simulink model "metareasoning"  (R2020a)
settings: Solver=FixedStepAuto  StartTime=0.0  StopTime=1000  FixedStep=0.5  RelTol=1e-3
PreLoadFcn:
  | Metareasoningpreloadfcn
InitFcn:
  | MetareasoningInitFcn
StopFcn:
  | trajectory_plot
values from neighbouring files (symbols this model uses):
  Clmax = 2.0    (= 2)    [Metareasoningpreloadfcn.m]
  Clmin = -.5    (= -0.5)    [Metareasoningpreloadfcn.m]
  g = 9.81    [Metareasoningpreloadfcn.m]
  goal_pos = [9000, 1E6, 0; -1E6, 23150+9000, 0]    [MetareasoningInitFcn.m]
  LOS_m = 9260    [Metareasoningpreloadfcn.m]
  num_ac = 2    [MetareasoningInitFcn.m]
  omega_chi = .2    (= 0.2)    [Metareasoningpreloadfcn.m]
  omega_gamma = .2    (= 0.2)    [Metareasoningpreloadfcn.m]
  omega_v = .3    (= 0.3)    [Metareasoningpreloadfcn.m]
  rho = 1.225    [Metareasoningpreloadfcn.m]
  S = 37.161    [Metareasoningpreloadfcn.m]
  tau_b = .5    (= 0.5)    [Metareasoningpreloadfcn.m]
  tau_n = .5    (= 0.5)    [Metareasoningpreloadfcn.m]
  tau_t = 1    [Metareasoningpreloadfcn.m]
  thrust_ic = 0.5*rho.*vel_ic.^2*S.*Cd    [MetareasoningInitFcn.m]
  Tmax = 25600*4.44822    (= 113874.432)    [Metareasoningpreloadfcn.m]
  W = 14515    [Metareasoningpreloadfcn.m]
undefined symbols (not defined in the file or in its folder): turnangles
libraries: asbswarm_lib x2, aerolibptmass x2, simulink x1
(part 1 of 3)
settings Model: Creator=Aidan  LastModifiedBy=Aidan

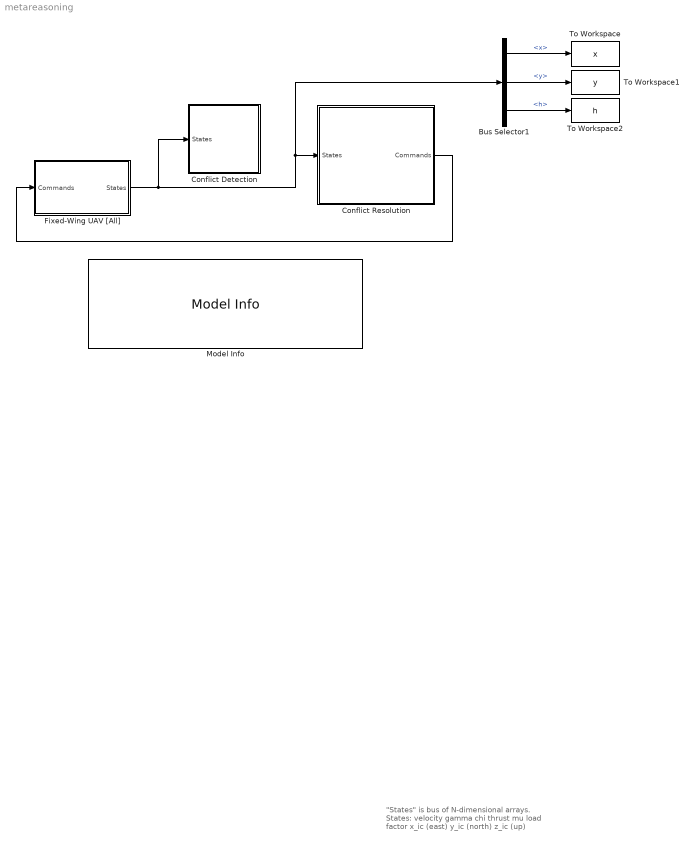
== system metareasoning ==
  note: "States" is bus of N-dimensional arrays.
      |
      | States:
      | velocity
      | gamma
      | chi
      | thrust
      | mu
      | load factor
      | x_ic (east)
      | y_ic (north)
      | z_ic (up)
  Bus Selector1 : BusSelector  OutputSignals=x,y,h
  Conflict Detection : Subsystem
      mask Display: image('C:\Users\Aidan\Downloads\exclamation_mark.png'); % Use "Edit Image" on toolstrip to change.
  Conflict Resolution : Subsystem
  Fixed-Wing UAV [All] : Subsystem
  Model Info : simulink/Model-Wide Utilities/Model Info  Frame=on  DisplayStringWithTags=|  HorizontalTextAlignment=Center  LeftAlignmentValue=0.5
      | Aidan Wallace
      | University of Maryland, College Park
      | 
      | This multiple-aircraft model is used to demonstrate the performance 
      | of various conflict detection and resolution methods for winged aircraft.
      | 
      | Fixed-Wing UAV and DynInversionControl blocks modified from Simulink
      | example model 'asbswarm'
      | 
      | %<LastModificationDate>
  To Workspace : ToWorkspace  VariableName=x  SaveFormat=Timeseries  SampleTime=-1
  To Workspace1 : ToWorkspace  VariableName=y  SaveFormat=Timeseries  SampleTime=-1
  To Workspace2 : ToWorkspace  VariableName=h  SaveFormat=Timeseries  SampleTime=-1
  wires:
  Bus Selector1/2 -> To Workspace1/1  "<y>"
  Bus Selector1/1 -> To Workspace/1  "<x>"
  Bus Selector1/3 -> To Workspace2/1  "<h>"
  Fixed-Wing UAV [All]/1(States) -> Bus Selector1/1, Conflict Resolution/1(States), Conflict Detection/1(States)
  Conflict Resolution/1(Commands) -> Fixed-Wing UAV [All]/1(Commands)

== system metareasoning/Conflict Detection ==
  States : Inport
  Bus Selector : BusSelector  OutputSignals=Velocity,chi,x,y
  State-Based Conflict Detection (Single Agent) : Subsystem  TreatAsAtomicUnit=on
  To Workspace : ToWorkspace  VariableName=tlos  SaveFormat=Timeseries  SampleTime=-1
  To Workspace1 : ToWorkspace  VariableName=tcpa  SaveFormat=Timeseries  SampleTime=-1
  wires:
  Bus Selector/2 -> State-Based Conflict Detection (Single Agent)/6(chi [all]), State-Based Conflict Detection (Single Agent)/2(chi (own))  "<chi>"
  Bus Selector/1 -> State-Based Conflict Detection (Single Agent)/1(Velocity (own)), State-Based Conflict Detection (Single Agent)/5(velocity [all])  "<Velocity>"
  Bus Selector/4 -> State-Based Conflict Detection (Single Agent)/8(y [all]), State-Based Conflict Detection (Single Agent)/4(y (own))  "<y>"
  State-Based Conflict Detection (Single Agent)/1(tlos) -> To Workspace/1  "tlos"
  Bus Selector/3 -> State-Based Conflict Detection (Single Agent)/7(x [all]), State-Based Conflict Detection (Single Agent)/3(x (own))  "<x>"
  States/1 -> Bus Selector/1
  State-Based Conflict Detection (Single Agent)/2(tcpa) -> To Workspace1/1

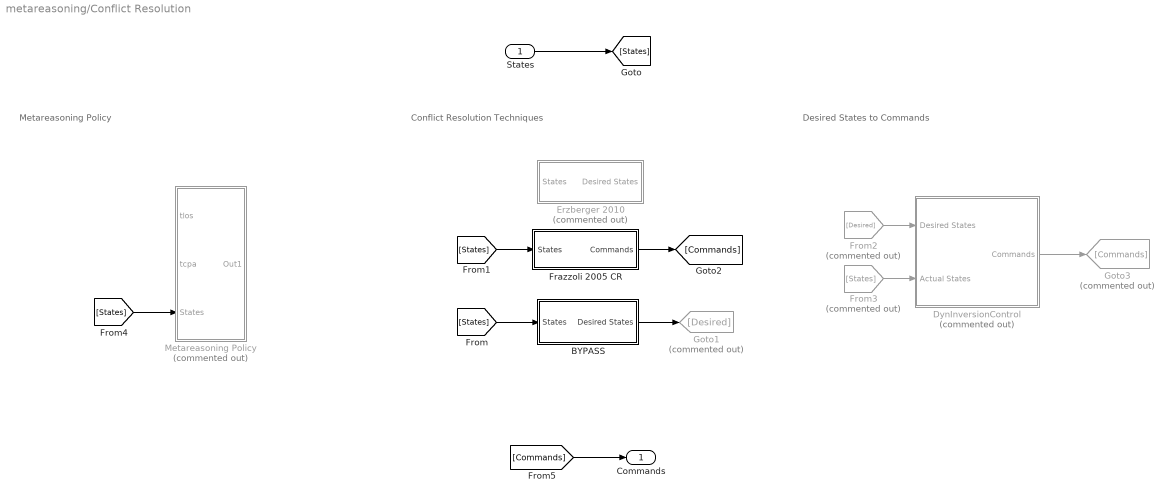
== system metareasoning/Conflict Resolution ==
  note: Desired States to Commands
  note: Conflict Resolution Techniques
  note: Metareasoning Policy
  States : Inport
  BYPASS : Subsystem
  DynInversionControl : Subsystem  Commented=on
  Erzberger 2010 : Subsystem  Commented=on
  Frazzoli 2005 CR : Subsystem
  From2 : From  Commented=on  GotoTag=Desired
  From3 : From  Commented=on  GotoTag=States
  Goto1 : Goto  Commented=on  GotoTag=Desired
  Goto3 : Goto  Commented=on  GotoTag=Commands
  Metareasoning Policy : Subsystem  Commented=on
  Commands : Outport
  wires:
  DynInversionControl/1(Commands) -> Goto3/1
  BYPASS/1(Desired States) -> Goto1/1
  States/1 -> [States]
  [States] -> BYPASS/1(States)
  [States] -> Frazzoli 2005 CR/1(States)
  From2/1 -> DynInversionControl/1(Desired States)
  From3/1 -> DynInversionControl/2(Actual States)
  [States] -> Metareasoning Policy/3(States)
  Frazzoli 2005 CR/1(Commands) -> [Commands]
  [Commands] -> Commands/1

== system metareasoning/Fixed-Wing UAV [All] ==
  Commands : Inport
  6DOF Point Mass (Coordinated Flight) : aerolibptmass/6th Order Point Mass (Coordinated Flight)  units=Metric (MKS)  gamma0=gamma_ic  chi0=chi_ic  V0=vel_ic  x0=x0  y0=y0  h0=h0  mass0=W/g
      settings: SourceProductBaseCode=AE
  6DOF Point Mass Forces (Coordinated Flight) : aerolibptmass/6th Order Point Mass Forces (Coordinated Flight)
      settings: SourceProductBaseCode=AE
  "Commands " : InportShadow
  EOM : Subsystem
  Integrator : Integrator  InitialCondition=[thrust_ic; zeros(1,num_ac); ones(1,num_ac)]
  Subsystem1 : Subsystem
  "V, gamma, chi2" : BusSelector  OutputSignals=gamma
  "V, gamma, chi4" : BusSelector  OutputSignals=mu
  alpha : Constant  Value=0
  makebus1 : Subsystem
  States : Outport  VectorParamsAs1DForOutWhenUnconnected=off
  wires:
  EOM/1(State Rates) -> Integrator/1
  Integrator/1 -> makebus1/1(In1)
  6DOF Point Mass Forces (Coordinated Flight)/2 -> 6DOF Point Mass (Coordinated Flight)/2
  6DOF Point Mass (Coordinated Flight)/3 -> makebus1/4(Velocity)
  6DOF Point Mass (Coordinated Flight)/1 -> makebus1/2(gamma)
  6DOF Point Mass Forces (Coordinated Flight)/1 -> 6DOF Point Mass (Coordinated Flight)/1
  6DOF Point Mass (Coordinated Flight)/2 -> makebus1/3(chi)
  6DOF Point Mass (Coordinated Flight)/6 -> makebus1/7(h)
  makebus1/1(Out2) -> States/1, "V, gamma, chi4"/1, "V, gamma, chi2"/1, Subsystem1/2(States), EOM/1(States)
  6DOF Point Mass Forces (Coordinated Flight)/3 -> 6DOF Point Mass (Coordinated Flight)/3
  Subsystem1/4(Thrust) -> 6DOF Point Mass Forces (Coordinated Flight)/4
  Subsystem1/2(Drag) -> 6DOF Point Mass Forces (Coordinated Flight)/2
  Subsystem1/1(Lift) -> 6DOF Point Mass Forces (Coordinated Flight)/1
  Subsystem1/3(Weight) -> 6DOF Point Mass Forces (Coordinated Flight)/3
  alpha/1 -> 6DOF Point Mass Forces (Coordinated Flight)/7
  "V, gamma, chi4"/1 -> 6DOF Point Mass Forces (Coordinated Flight)/6  "<mu>"
  6DOF Point Mass (Coordinated Flight)/4 -> makebus1/5(x)
  6DOF Point Mass (Coordinated Flight)/5 -> makebus1/6(y)
  "Commands "/1 -> Subsystem1/1(Cmd)
  Commands/1 -> EOM/2(Commands)
  "V, gamma, chi2"/1 -> 6DOF Point Mass Forces (Coordinated Flight)/5  "<gamma>"

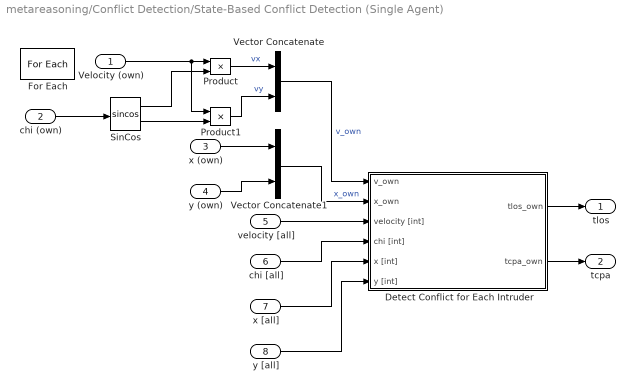
== system metareasoning/Conflict Detection/State-Based Conflict Detection (Single Agent) ==
  Velocity (own) : Inport  Partition=on  PartitionDimension=1  PartitionWidth=1  PartitionOffset=0
  chi (own) : Inport  Port=2  Partition=on  PartitionDimension=1  PartitionWidth=1  PartitionOffset=0
  x (own) : Inport  Port=3  Partition=on  PartitionDimension=1  PartitionWidth=1  PartitionOffset=0
  y (own) : Inport  Port=4  Partition=on  PartitionDimension=1  PartitionWidth=1  PartitionOffset=0
  velocity [all] : Inport  Port=5
  chi [all] : Inport  Port=6
  x [all] : Inport  Port=7
  y [all] : Inport  Port=8
  Detect Conflict for Each Intruder : Subsystem  TreatAsAtomicUnit=on
  For Each : ForEach  DisableCoverage=on
  Product : Product
  Product1 : Product
  SinCos : Trigonometry  Operator=sincos
  Vector Concatenate : Concatenate
  Vector Concatenate1 : Concatenate
  tlos : Outport  ConcatenationDimension=1
  tcpa : Outport  Port=2  ConcatenationDimension=1
  wires:
  Product1/1 -> Vector Concatenate/2  "vy"
  SinCos/1 -> Product/2
  Detect Conflict for Each Intruder/2(tcpa_own) -> tcpa/1
  Vector Concatenate/1 -> Detect Conflict for Each Intruder/1(v_own)  "v_own"
  Vector Concatenate1/1 -> Detect Conflict for Each Intruder/2(x_own)  "x_own"
  Detect Conflict for Each Intruder/1(tlos_own) -> tlos/1
  chi (own)/1 -> SinCos/1
  chi [all]/1 -> Detect Conflict for Each Intruder/4(chi [int])
  y [all]/1 -> Detect Conflict for Each Intruder/6(y [int])
  x [all]/1 -> Detect Conflict for Each Intruder/5(x [int])
  velocity [all]/1 -> Detect Conflict for Each Intruder/3(velocity [int])
  Product/1 -> Vector Concatenate/1  "vx"
  SinCos/2 -> Product1/2
  y (own)/1 -> Vector Concatenate1/2
  x (own)/1 -> Vector Concatenate1/1
  Velocity (own)/1 -> Product/1, Product1/1

== system metareasoning/Conflict Resolution/BYPASS ==
  States : Inport
  Bus Creator : BusCreator  Inputs=3
  Bus Selector : BusSelector  OutputSignals=Velocity,gamma,chi
  Sum : Sum  Inputs=|++
  Sum1 : Sum  Inputs=|++
  Sum2 : Sum  Inputs=|++
  Zero : Constant  Value=0  OutDataTypeStr=Inherit: Inherit via back propagation
  Desired States : Outport
  wires:
  States/1 -> Bus Selector/1
  Bus Creator/1 -> Desired States/1
  Bus Selector/1 -> Sum/1  "<Velocity>"
  Bus Selector/2 -> Sum1/1  "<gamma>"
  Zero/1 -> Sum2/2, Sum1/2, Sum/2
  Bus Selector/3 -> Sum2/1  "<chi>"
  Sum2/1 -> Bus Creator/3  "chi_desired"
  Sum1/1 -> Bus Creator/2  "gamma_desired"
  Sum/1 -> Bus Creator/1  "Velocity_desired"

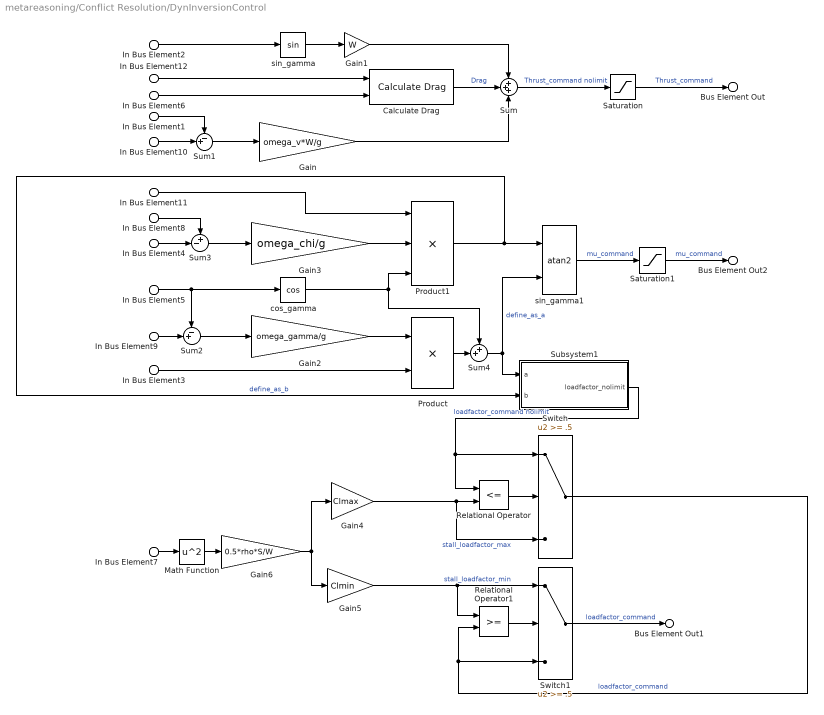
== system metareasoning/Conflict Resolution/DynInversionControl ==
  In Bus Element8 : Inport  PortName=Desired States  Element=chi_desired
  In Bus Element9 : Inport  PortName=Desired States  Element=gamma_desired
  In Bus Element10 : Inport  PortName=Desired States  Element=Velocity_desired
  In Bus Element{1,3,7,11..12} (5 alike) : Inport  Port=2  PortName=Actual States  Element=Velocity
  In Bus Element5 : Inport  Port=2  PortName=Actual States  Element=gamma
  In Bus Element2 : Inport  Port=2  PortName=Actual States  Element=gamma
  In Bus Element4 : Inport  Port=2  PortName=Actual States  Element=chi
  In Bus Element6 : Inport  Port=2  PortName=Actual States  Element=loadfactor
  Calculate Drag : asbswarm_lib/Calculate Drag  SystemSampleTime=-1  Latency=0  AutoFrameSizeCalculation=off
      settings: SourceProductBaseCode=AE
  Gain : Gain  Gain=omega_v*W/g  SaturateOnIntegerOverflow=on  OutDataTypeStr=Inherit: Same as input  ParamDataTypeStr=Inherit: Same as input
  Gain1 : Gain  Gain=W  SaturateOnIntegerOverflow=on  OutDataTypeStr=Inherit: Same as input  ParamDataTypeStr=Inherit: Same as input
  Gain2 : Gain  Gain=omega_gamma/g  SaturateOnIntegerOverflow=on  OutDataTypeStr=Inherit: Same as input  ParamDataTypeStr=Inherit: Same as input
  Gain3 : Gain  Gain=omega_chi/g  SaturateOnIntegerOverflow=on  OutDataTypeStr=Inherit: Same as input  ParamDataTypeStr=Inherit: Same as input
  Gain4 : Gain  Gain=Clmax  SaturateOnIntegerOverflow=on  OutDataTypeStr=Inherit: Same as input  ParamDataTypeStr=Inherit: Same as input
  Gain5 : Gain  Gain=Clmin  SaturateOnIntegerOverflow=on  OutDataTypeStr=Inherit: Same as input  ParamDataTypeStr=Inherit: Same as input
  Gain6 : Gain  Gain=0.5*rho*S/W  SaturateOnIntegerOverflow=on  OutDataTypeStr=Inherit: Same as input  ParamDataTypeStr=Inherit: Same as input
  Math Function : Math  Operator=square  SignedPower=on  SaturateOnIntegerOverflow=on
  Product : Product  InputSameDT=on  SaturateOnIntegerOverflow=on  OutDataTypeStr=Inherit: Same as first input
  Product1 : Product  Inputs=3  InputSameDT=on  SaturateOnIntegerOverflow=on  OutDataTypeStr=Inherit: Same as first input
  Relational Operator : RelationalOperator  Operator=<=  RndMeth=Nearest  InputSameDT=on
  Relational Operator1 : RelationalOperator  RndMeth=Nearest  InputSameDT=on
  Saturation : Saturate  UpperLimit=Tmax  LowerLimit=0
  Saturation1 : Saturate  UpperLimit=pi/2  LowerLimit=-pi/2
  Subsystem1 : Subsystem
  Sum : Sum  Inputs=+++  InputSameDT=on  SaturateOnIntegerOverflow=on  OutDataTypeStr=Inherit: Same as first input
  Sum1 : Sum  Inputs=-+|  InputSameDT=on  SaturateOnIntegerOverflow=on  OutDataTypeStr=Inherit: Same as first input
  Sum2 : Sum  Inputs=-+|  InputSameDT=on  SaturateOnIntegerOverflow=on  OutDataTypeStr=Inherit: Same as first input
  Sum3 : Sum  Inputs=+-|  InputSameDT=on  SaturateOnIntegerOverflow=on  OutDataTypeStr=Inherit: Same as first input
  Sum4 : Sum  Inputs=++|  InputSameDT=on  SaturateOnIntegerOverflow=on  OutDataTypeStr=Inherit: Same as first input
  Switch : Switch  Threshold=.5  SaturateOnIntegerOverflow=on  InputSameDT=on
  Switch1 : Switch  Threshold=.5  SaturateOnIntegerOverflow=on  InputSameDT=on
  cos_gamma : Trigonometry  Operator=cos
  sin_gamma : Trigonometry
  sin_gamma1 : Trigonometry  Operator=atan2
  Bus Element Out : Outport  VectorParamsAs1DForOutWhenUnconnected=off  PortName=Commands  Element=Thrust_command
  Bus Element Out1 : Outport  VectorParamsAs1DForOutWhenUnconnected=off  PortName=Commands  Element=loadfactor_command
  Bus Element Out2 : Outport  VectorParamsAs1DForOutWhenUnconnected=off  PortName=Commands  Element=mu_command
  wires:
  In Bus Element9/1 -> Sum2/2
  In Bus Element6/1 -> Calculate Drag/2
  In Bus Element1/1 -> Sum1/1
  In Bus Element10/1 -> Sum1/2
  Sum1/1 -> Gain/1
  Calculate Drag/1 -> Sum/2  "Drag"
  Gain/1 -> Sum/3
  In Bus Element2/1 -> sin_gamma/1
  sin_gamma/1 -> Gain1/1
  Gain1/1 -> Sum/1
  Sum/1 -> Saturation/1  "Thrust_command nolimit"
  In Bus Element5/1 -> Sum2/1, cos_gamma/1
  In Bus Element8/1 -> Sum3/1
  In Bus Element4/1 -> Sum3/2
  Sum2/1 -> Gain2/1
  Gain2/1 -> Product/1
  In Bus Element3/1 -> Product/2
  Product/1 -> Sum4/2
  cos_gamma/1 -> Product1/3, Sum4/1
  Sum4/1 -> Subsystem1/1(a), sin_gamma1/2  "define_as_a"
  Sum3/1 -> Gain3/1
  Product1/1 -> Subsystem1/2(b), sin_gamma1/1  "define_as_b"
  sin_gamma1/1 -> Saturation1/1  "mu_command"
  Subsystem1/1(loadfactor_nolimit) -> Switch/1, Relational Operator/1  "loadfactor_command nolimit"
  Saturation/1 -> Bus Element Out/1  "Thrust_command"
  In Bus Element7/1 -> Math Function/1
  Gain3/1 -> Product1/2
  Gain4/1 -> Switch/3, Relational Operator/2  "stall_loadfactor_max"
  Relational Operator/1 -> Switch/2
  Math Function/1 -> Gain6/1
  Saturation1/1 -> Bus Element Out2/1  "mu_command"
  Gain5/1 -> Switch1/1, Relational Operator1/1  "stall_loadfactor_min"
  Switch/1 -> Switch1/3, Relational Operator1/2  "loadfactor_command"
  Relational Operator1/1 -> Switch1/2
  Switch1/1 -> Bus Element Out1/1  "loadfactor_command"
  In Bus Element11/1 -> Product1/1
  In Bus Element12/1 -> Calculate Drag/1
  Gain6/1 -> Gain4/1, Gain5/1

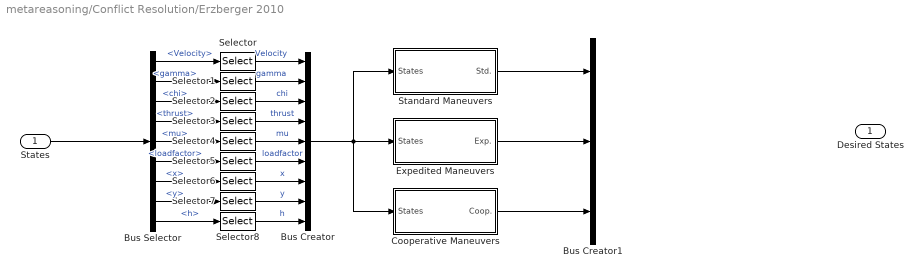
== system metareasoning/Conflict Resolution/Erzberger 2010 ==
  States : Inport
  Bus Creator : BusCreator  Inputs=9
  Bus Creator1 : BusCreator  Inputs=3
  Bus Selector : BusSelector  OutputSignals=Velocity,gamma,chi,thrust,mu,loadfactor,x,y,h
  Cooperative Maneuvers : Subsystem
  Expedited Maneuvers : Subsystem
  Selector{,1..8} (9 alike) : Selector  InputPortWidth=num_ac  IndexOptions=Index vector (dialog)  Indices=[1 2]  OutputSizes=1
  Standard Maneuvers : Subsystem
  Desired States : Outport
  wires:
  States/1 -> Bus Selector/1
  Bus Selector/1 -> Selector/1  "<Velocity>"
  Bus Selector/2 -> Selector1/1  "<gamma>"
  Bus Selector/3 -> Selector2/1  "<chi>"
  Bus Selector/4 -> Selector3/1  "<thrust>"
  Bus Selector/5 -> Selector4/1  "<mu>"
  Bus Selector/6 -> Selector5/1  "<loadfactor>"
  Bus Selector/7 -> Selector6/1  "<x>"
  Bus Selector/8 -> Selector7/1  "<y>"
  Bus Selector/9 -> Selector8/1  "<h>"
  Selector/1 -> Bus Creator/1  "Velocity"
  Selector1/1 -> Bus Creator/2  "gamma"
  Selector2/1 -> Bus Creator/3  "chi"
  Selector3/1 -> Bus Creator/4  "thrust"
  Selector4/1 -> Bus Creator/5  "mu"
  Selector5/1 -> Bus Creator/6  "loadfactor"
  Selector6/1 -> Bus Creator/7  "x"
  Selector7/1 -> Bus Creator/8  "y"
  Selector8/1 -> Bus Creator/9  "h"
  Bus Creator/1 -> Standard Maneuvers/1(States), Cooperative Maneuvers/1(States), Expedited Maneuvers/1(States)
  Standard Maneuvers/1(Std.) -> Bus Creator1/1
  Cooperative Maneuvers/1(Coop.) -> Bus Creator1/3
  Expedited Maneuvers/1(Exp.) -> Bus Creator1/2

== system metareasoning/Conflict Resolution/Frazzoli 2005 CR ==
  States : Inport
  Bus Selector : BusSelector  OutputSignals=x,y,chi,Velocity,thrust
  Constant : Constant  Value=goal_pos
  Single-Agent Planning : Subsystem  TreatAsAtomicUnit=on
  Bus Element Out : Outport  PortName=Commands  Element=Thrust_command
  Bus Element Out1 : Outport  PortName=Commands  Element=mu_command
  Bus Element Out2 : Outport  PortName=Commands  Element=loadfactor_command
  wires:
  States/1 -> Bus Selector/1
  Bus Selector/1 -> Single-Agent Planning/5(x [all]), Single-Agent Planning/1(<x>)  "<x>"
  Bus Selector/2 -> Single-Agent Planning/6(y [all]), Single-Agent Planning/2(<y>)  "<y>"
  Bus Selector/3 -> Single-Agent Planning/7(chi [all]), Single-Agent Planning/3(<chi>)  "<chi>"
  Single-Agent Planning/1(Thrust_command) -> Bus Element Out/1
  Constant/1 -> Single-Agent Planning/8(goal_pos)
  Bus Selector/4 -> Single-Agent Planning/4(Velocity)  "<Velocity>"
  Bus Selector/5 -> Single-Agent Planning/9(Thrust)  "<thrust>"
  Single-Agent Planning/2(mu_command) -> Bus Element Out1/1
  Single-Agent Planning/3(loadfactor_command) -> Bus Element Out2/1

== system metareasoning/Conflict Resolution/Metareasoning Policy ==
  tlos : Inport
  tcpa : Inport  Port=2
  States : Inport  Port=3
  Out1 : Outport
  wires:
  tlos/1 -> Out1/1

== system metareasoning/Fixed-Wing UAV [All]/EOM ==
  States : Inport
  Commands : Inport  Port=2
  Math Function : Math  Operator=transpose  SignedPower=on  SaturateOnIntegerOverflow=on
  Matrix Concatenation : Concatenate  NumInputs=3  Mode=Multidimensional array  ConcatenateDimension=2
  "[thrust_dot mu_dot loadfactor_dot]" : Subsystem
  State Rates : Outport  VectorParamsAs1DForOutWhenUnconnected=off
  wires:
  Commands/1 -> "[thrust_dot mu_dot loadfactor_dot]"/1(Commands)
  States/1 -> "[thrust_dot mu_dot loadfactor_dot]"/2(States)
  "[thrust_dot mu_dot loadfactor_dot]"/2(mu_dot) -> Matrix Concatenation/2
  "[thrust_dot mu_dot loadfactor_dot]"/1(thrust_dot) -> Matrix Concatenation/1
  "[thrust_dot mu_dot loadfactor_dot]"/3(loadfactor_dot) -> Matrix Concatenation/3
  Math Function/1 -> State Rates/1
  Matrix Concatenation/1 -> Math Function/1

== system metareasoning/Fixed-Wing UAV [All]/Subsystem1 ==
  Bus Element In2 : Inport  PortName=Cmd  Element=Thrust_command
  Bus Element In : Inport  Port=2  PortName=States  Element=loadfactor
  Bus Element In1 : Inport  Port=2  PortName=States  Element=loadfactor
  Bus Element In3 : Inport  Port=2  PortName=States  Element=Velocity
  Calculate Drag : asbswarm_lib/Calculate Drag  SystemSampleTime=-1  Latency=0  AutoFrameSizeCalculation=off
      settings: SourceProductBaseCode=AE
  Constant : Constant  Value=W
  Product1 : Product  RndMeth=Zero
  Lift : Outport  VectorParamsAs1DForOutWhenUnconnected=off
  Drag : Outport  Port=2  VectorParamsAs1DForOutWhenUnconnected=off
  Weight : Outport  Port=3  VectorParamsAs1DForOutWhenUnconnected=off
  Thrust : Outport  Port=4  VectorParamsAs1DForOutWhenUnconnected=off
  wires:
  Constant/1 -> Product1/2, Weight/1
  Calculate Drag/1 -> Drag/1
  Bus Element In2/1 -> Thrust/1
  Product1/1 -> Lift/1
  Bus Element In3/1 -> Calculate Drag/1
  Bus Element In/1 -> Calculate Drag/2
  Bus Element In1/1 -> Product1/1

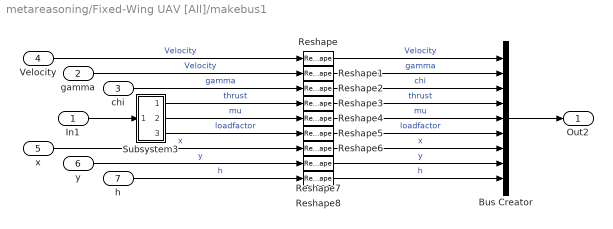
== system metareasoning/Fixed-Wing UAV [All]/makebus1 ==
  In1 : Inport  PortDimensions=[3,num_ac]
  gamma : Inport  Port=2  PortDimensions=[1,num_ac]
  chi : Inport  Port=3  PortDimensions=[1,num_ac]
  Velocity : Inport  Port=4  PortDimensions=[1,num_ac]
  x : Inport  Port=5  PortDimensions=[1,num_ac]
  y : Inport  Port=6  PortDimensions=[1,num_ac]
  h : Inport  Port=7  PortDimensions=[1,num_ac]
  Bus Creator : BusCreator  Inputs=9
  Reshape{,1..8} (9 alike) : Reshape
  Subsystem3 : Subsystem
      mask Display: disp('Select\nRows');
  Out2 : Outport  VectorParamsAs1DForOutWhenUnconnected=off
  wires:
  In1/1 -> Subsystem3/1(In1)
  Reshape8/1 -> Bus Creator/9  "h"
  Reshape7/1 -> Bus Creator/8  "y"
  Reshape6/1 -> Bus Creator/7  "x"
  Reshape5/1 -> Bus Creator/6  "loadfactor"
  Reshape4/1 -> Bus Creator/5  "mu"
  Reshape3/1 -> Bus Creator/4  "thrust"
  Reshape2/1 -> Bus Creator/3  "chi"
  Reshape1/1 -> Bus Creator/2  "gamma"
  Reshape/1 -> Bus Creator/1  "Velocity"
  Bus Creator/1 -> Out2/1
  h/1 -> Reshape8/1  "h"
  y/1 -> Reshape7/1  "y"
  x/1 -> Reshape6/1  "x"
  Subsystem3/3(Out3) -> Reshape5/1  "loadfactor"
  Subsystem3/2(Out2) -> Reshape4/1  "mu"
  Subsystem3/1(Out1) -> Reshape3/1  "thrust"
  chi/1 -> Reshape2/1  "gamma"
  gamma/1 -> Reshape1/1  "Velocity"
  Velocity/1 -> Reshape/1  "Velocity"

== system metareasoning/Conflict Detection/State-Based Conflict Detection (Single Agent)/Detect Conflict for Each Intruder ==
  v_own : Inport
  x_own : Inport  Port=2
  velocity [int] : Inport  Port=3  Partition=on  PartitionDimension=1  PartitionWidth=1  PartitionOffset=0
  chi [int] : Inport  Port=4  Partition=on  PartitionDimension=1  PartitionWidth=1  PartitionOffset=0
  x [int] : Inport  Port=5  Partition=on  PartitionDimension=1  PartitionWidth=1  PartitionOffset=0
  y [int] : Inport  Port=6  Partition=on  PartitionDimension=1  PartitionWidth=1  PartitionOffset=0
  Conflict Detection : MATLAB Function  TreatAsAtomicUnit=on
  Constant : Constant  Value=LOS_m
  For Each : ForEach  DisableCoverage=on
  Product : Product
  Product1 : Product
  SinCos : Trigonometry  Operator=sincos
  Vector Concatenate : Concatenate
  Vector Concatenate1 : Concatenate
  tlos_own : Outport  ConcatenationDimension=2
  tcpa_own : Outport  Port=2  ConcatenationDimension=2
  wires:
  velocity [int]/1 -> Product/1, Product1/1
  Product/1 -> Vector Concatenate/1  "vx"
  x_own/1 -> Conflict Detection/2(x_own)
  Constant/1 -> Conflict Detection/5(LOS_m)
  Conflict Detection/1(tlos) -> tlos_own/1
  chi [int]/1 -> SinCos/1
  y [int]/1 -> Vector Concatenate1/2
  v_own/1 -> Conflict Detection/1(v_own)
  SinCos/1 -> Product/2
  Vector Concatenate/1 -> Conflict Detection/3(v_int)  "v_int"
  SinCos/2 -> Product1/2
  Vector Concatenate1/1 -> Conflict Detection/4(x_int)  "x_int"
  Conflict Detection/2(tcpa) -> tcpa_own/1
  Product1/1 -> Vector Concatenate/2  "vy"
  x [int]/1 -> Vector Concatenate1/1

== system metareasoning/Conflict Resolution/DynInversionControl/Subsystem1 ==
  a : Inport
  b : Inport  Port=2
  Math Function : Math  Operator=square  SignedPower=on  SaturateOnIntegerOverflow=on
  Math Function1 : Math  Operator=square  SignedPower=on  SaturateOnIntegerOverflow=on
  Sqrt : Sqrt  SaturateOnIntegerOverflow=on
  Sum : Sum  Inputs=|++  InputSameDT=on  SaturateOnIntegerOverflow=on  OutDataTypeStr=Inherit: Same as first input
  loadfactor_nolimit : Outport  VectorParamsAs1DForOutWhenUnconnected=off
  wires:
  Sqrt/1 -> loadfactor_nolimit/1
  Math Function1/1 -> Sum/2
  Math Function/1 -> Sum/1
  b/1 -> Math Function1/1
  a/1 -> Math Function/1
  Sum/1 -> Sqrt/1

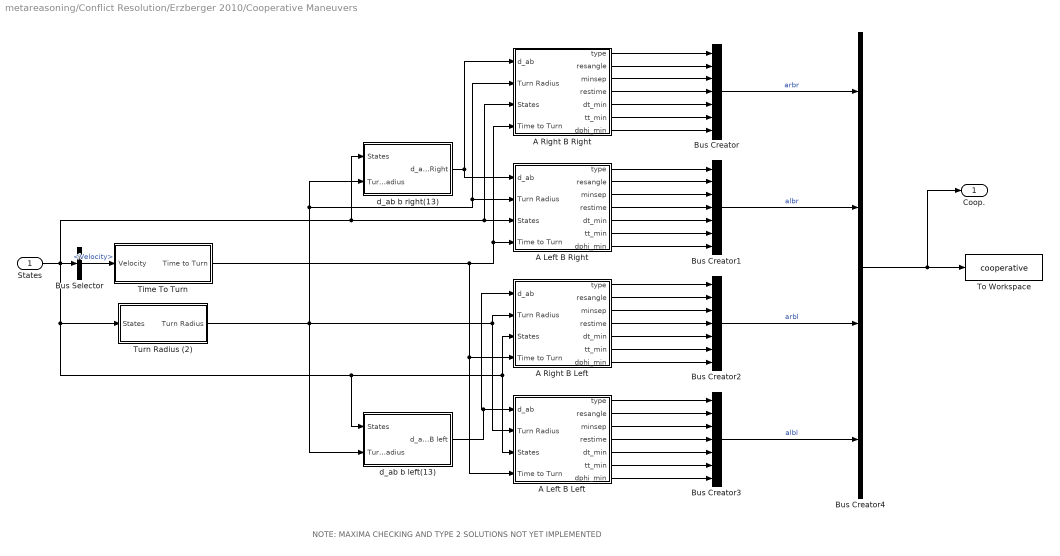
== system metareasoning/Conflict Resolution/Erzberger 2010/Cooperative Maneuvers ==
  note: NOTE: MAXIMA CHECKING AND TYPE 2 SOLUTIONS NOT YET IMPLEMENTED
  States : Inport
  A Left B Left : Subsystem
  A Left B Right : Subsystem
  A Right B Left : Subsystem
  A Right B Right : Subsystem
  Bus Creator{,1..3} (4 alike) : BusCreator  Inputs=7
  Bus Creator4 : BusCreator  Inputs=4
  Bus Selector : BusSelector  OutputSignals=Velocity
  Time To Turn : Subsystem
  To Workspace : ToWorkspace  VariableName=cooperative  SaveFormat=Timeseries  SampleTime=-1
  Turn Radius (2) : Subsystem
  d_ab b left(13) : Subsystem
  d_ab b right(13) : Subsystem
  Coop. : Outport
  wires:
  Bus Selector/1 -> Time To Turn/1(Velocity)  "<Velocity>"
  States/1 -> A Right B Left/3(States), A Left B Left/3(States), d_ab b left(13)/1(States), Turn Radius (2)/1(States), d_ab b right(13)/1(States), A Right B Right/3(States), A Left B Right/3(States), Bus Selector/1
  Time To Turn/1(Time to Turn) -> A Right B Left/4(Time to Turn), A Left B Left/4(Time to Turn), A Left B Right/4(Time to Turn), A Right B Right/4(Time to Turn)
  Turn Radius (2)/1(Turn Radius) -> d_ab b left(13)/2(Turn Radius), A Right B Left/2(Turn Radius), A Left B Left/2(Turn Radius), d_ab b right(13)/2(Turn Radius), A Left B Right/2(Turn Radius), A Right B Right/2(Turn Radius)
  d_ab b right(13)/1(d_ab B Right) -> A Left B Right/1(d_ab), A Right B Right/1(d_ab)
  A Right B Right/2(resangle) -> Bus Creator/2
  A Right B Right/3(minsep) -> Bus Creator/3
  A Right B Right/4(restime) -> Bus Creator/4
  A Right B Right/5(dt_min) -> Bus Creator/5
  A Right B Right/6(tt_min) -> Bus Creator/6
  A Right B Right/7(dphi_min) -> Bus Creator/7
  A Right B Right/1(type) -> Bus Creator/1
  Bus Creator/1 -> Bus Creator4/1  "arbr"
  Bus Creator1/1 -> Bus Creator4/2  "albr"
  Bus Creator2/1 -> Bus Creator4/3  "arbl"
  Bus Creator3/1 -> Bus Creator4/4  "albl"
  Bus Creator4/1 -> Coop./1, To Workspace/1
  A Left B Right/2(resangle) -> Bus Creator1/2
  A Left B Right/1(type) -> Bus Creator1/1
  A Left B Right/3(minsep) -> Bus Creator1/3
  A Left B Right/4(restime) -> Bus Creator1/4
  A Left B Right/5(dt_min) -> Bus Creator1/5
  A Left B Right/6(tt_min) -> Bus Creator1/6
  A Left B Right/7(dphi_min) -> Bus Creator1/7
  A Left B Left/1(type) -> Bus Creator3/1
  A Left B Left/2(resangle) -> Bus Creator3/2
  A Left B Left/3(minsep) -> Bus Creator3/3
  A Left B Left/4(restime) -> Bus Creator3/4
  A Left B Left/5(dt_min) -> Bus Creator3/5
  A Left B Left/6(tt_min) -> Bus Creator3/6
  A Left B Left/7(dphi_min) -> Bus Creator3/7
  d_ab b left(13)/1(d_ab B left) -> A Right B Left/1(d_ab), A Left B Left/1(d_ab)
  A Right B Left/1(type) -> Bus Creator2/1
  A Right B Left/2(resangle) -> Bus Creator2/2
  A Right B Left/3(minsep) -> Bus Creator2/3
  A Right B Left/4(restime) -> Bus Creator2/4
  A Right B Left/5(dt_min) -> Bus Creator2/5
  A Right B Left/6(tt_min) -> Bus Creator2/6
  A Right B Left/7(dphi_min) -> Bus Creator2/7

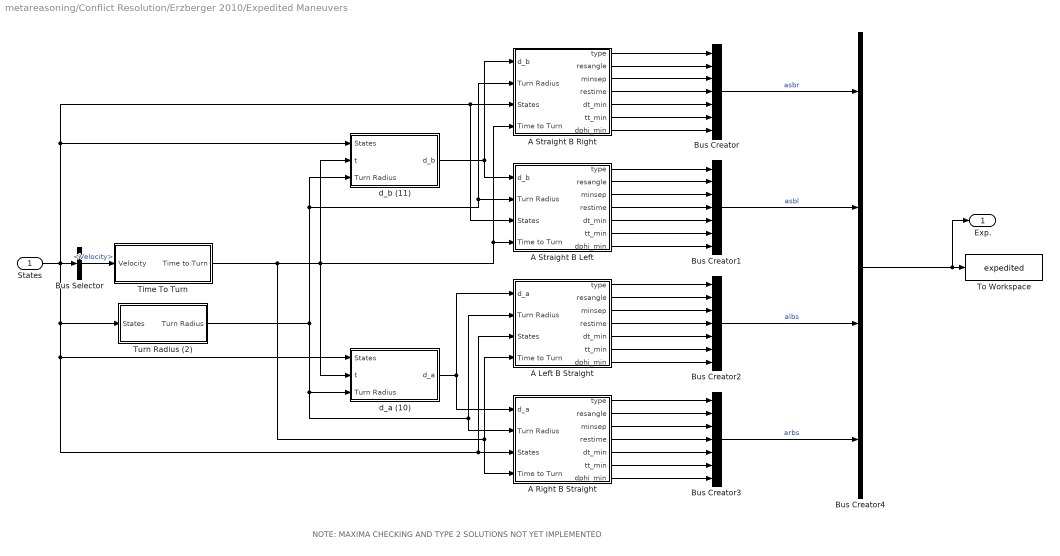
== system metareasoning/Conflict Resolution/Erzberger 2010/Expedited Maneuvers ==
  note: NOTE: MAXIMA CHECKING AND TYPE 2 SOLUTIONS NOT YET IMPLEMENTED
  States : Inport
  A Left B Straight : Subsystem
  A Right B Straight : Subsystem
  A Straight B Left : Subsystem
  A Straight B Right : Subsystem
  Bus Creator{,1..3} (4 alike) : BusCreator  Inputs=7
  Bus Creator4 : BusCreator  Inputs=4
  Bus Selector : BusSelector  OutputSignals=Velocity
  Time To Turn : Subsystem
  To Workspace : ToWorkspace  VariableName=expedited  SaveFormat=Timeseries  SampleTime=-1
  Turn Radius (2) : Subsystem
  d_a (10) : Subsystem
  d_b (11) : Subsystem
  Exp. : Outport
  wires:
  Bus Selector/1 -> Time To Turn/1(Velocity)  "<Velocity>"
  d_a (10)/1(d_a) -> A Left B Straight/1(d_a), A Right B Straight/1(d_a)
  States/1 -> d_a (10)/1(States), A Left B Straight/3(States), A Right B Straight/3(States), Turn Radius (2)/1(States), A Straight B Left/3(States), A Straight B Right/3(States), d_b (11)/1(States), Bus Selector/1
  Time To Turn/1(Time to Turn) -> d_b (11)/2(t), A Straight B Right/4(Time to Turn), A Straight B Left/4(Time to Turn), d_a (10)/2(t), A Left B Straight/4(Time to Turn), A Right B Straight/4(Time to Turn)
  Turn Radius (2)/1(Turn Radius) -> d_b (11)/3(Turn Radius), A Straight B Left/2(Turn Radius), A Straight B Right/2(Turn Radius), A Left B Straight/2(Turn Radius), A Right B Straight/2(Turn Radius), d_a (10)/3(Turn Radius)
  d_b (11)/1(d_b) -> A Straight B Right/1(d_b), A Straight B Left/1(d_b)
  A Straight B Right/2(resangle) -> Bus Creator/2
  A Straight B Right/3(minsep) -> Bus Creator/3
  A Straight B Right/4(restime) -> Bus Creator/4
  A Straight B Right/5(dt_min) -> Bus Creator/5
  A Straight B Right/6(tt_min) -> Bus Creator/6
  A Straight B Right/7(dphi_min) -> Bus Creator/7
  A Straight B Right/1(type) -> Bus Creator/1
  Bus Creator/1 -> Bus Creator4/1  "asbr"
  A Straight B Left/7(dphi_min) -> Bus Creator1/7
  A Straight B Left/6(tt_min) -> Bus Creator1/6
  Bus Creator1/1 -> Bus Creator4/2  "asbl"
  A Straight B Left/3(minsep) -> Bus Creator1/3
  A Straight B Left/5(dt_min) -> Bus Creator1/5
  A Straight B Left/1(type) -> Bus Creator1/1
  A Straight B Left/2(resangle) -> Bus Creator1/2
  A Straight B Left/4(restime) -> Bus Creator1/4
  A Left B Straight/7(dphi_min) -> Bus Creator2/7
  A Left B Straight/6(tt_min) -> Bus Creator2/6
  Bus Creator2/1 -> Bus Creator4/3  "albs"
  A Left B Straight/3(minsep) -> Bus Creator2/3
  A Left B Straight/5(dt_min) -> Bus Creator2/5
  A Left B Straight/1(type) -> Bus Creator2/1
  A Left B Straight/2(resangle) -> Bus Creator2/2
  A Left B Straight/4(restime) -> Bus Creator2/4
  A Right B Straight/7(dphi_min) -> Bus Creator3/7
  A Right B Straight/6(tt_min) -> Bus Creator3/6
  Bus Creator3/1 -> Bus Creator4/4  "arbs"
  A Right B Straight/3(minsep) -> Bus Creator3/3
  A Right B Straight/5(dt_min) -> Bus Creator3/5
  A Right B Straight/1(type) -> Bus Creator3/1
  A Right B Straight/2(resangle) -> Bus Creator3/2
  A Right B Straight/4(restime) -> Bus Creator3/4
  Bus Creator4/1 -> Exp./1, To Workspace/1

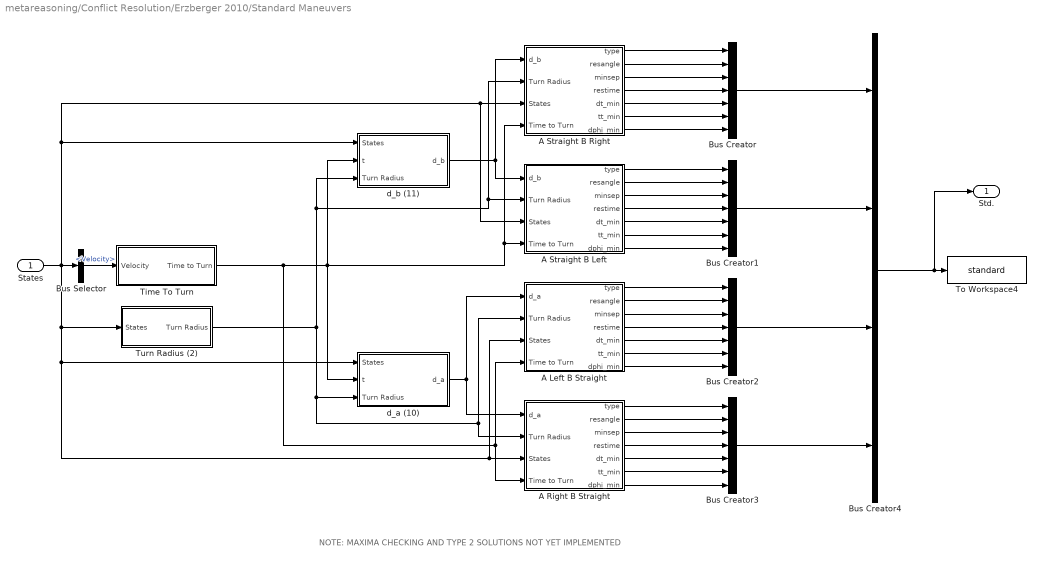
== system metareasoning/Conflict Resolution/Erzberger 2010/Standard Maneuvers ==
  note: NOTE: MAXIMA CHECKING AND TYPE 2 SOLUTIONS NOT YET IMPLEMENTED
  States : Inport
  A Left B Straight : Subsystem
  A Right B Straight : Subsystem
  A Straight B Left : Subsystem
  A Straight B Right : Subsystem
  Bus Creator{,1..3} (4 alike) : BusCreator  Inputs=7
  Bus Creator4 : BusCreator  Inputs=4
  Bus Selector : BusSelector  OutputSignals=Velocity
  Time To Turn : Subsystem
  To Workspace4 : ToWorkspace  VariableName=standard  SaveFormat=Timeseries  SampleTime=-1
  Turn Radius (2) : Subsystem
  d_a (10) : Subsystem
  d_b (11) : Subsystem
  Std. : Outport
  wires:
  Bus Selector/1 -> Time To Turn/1(Velocity)  "<Velocity>"
  d_a (10)/1(d_a) -> A Left B Straight/1(d_a), A Right B Straight/1(d_a)
  States/1 -> d_a (10)/1(States), A Left B Straight/3(States), A Right B Straight/3(States), Turn Radius (2)/1(States), A Straight B Left/3(States), A Straight B Right/3(States), d_b (11)/1(States), Bus Selector/1
  Time To Turn/1(Time to Turn) -> d_b (11)/2(t), A Straight B Right/4(Time to Turn), A Straight B Left/4(Time to Turn), d_a (10)/2(t), A Left B Straight/4(Time to Turn), A Right B Straight/4(Time to Turn)
  Turn Radius (2)/1(Turn Radius) -> d_b (11)/3(Turn Radius), A Straight B Left/2(Turn Radius), A Straight B Right/2(Turn Radius), A Left B Straight/2(Turn Radius), A Right B Straight/2(Turn Radius), d_a (10)/3(Turn Radius)
  d_b (11)/1(d_b) -> A Straight B Right/1(d_b), A Straight B Left/1(d_b)
  A Straight B Right/2(resangle) -> Bus Creator/2
  A Straight B Right/3(minsep) -> Bus Creator/3
  A Straight B Right/4(restime) -> Bus Creator/4
  A Straight B Right/5(dt_min) -> Bus Creator/5
  A Straight B Right/6(tt_min) -> Bus Creator/6
  A Straight B Right/7(dphi_min) -> Bus Creator/7
  A Straight B Right/1(type) -> Bus Creator/1
  Bus Creator/1 -> Bus Creator4/1
  A Straight B Left/7(dphi_min) -> Bus Creator1/7
  A Straight B Left/6(tt_min) -> Bus Creator1/6
  Bus Creator1/1 -> Bus Creator4/2
  A Straight B Left/3(minsep) -> Bus Creator1/3
  A Straight B Left/5(dt_min) -> Bus Creator1/5
  A Straight B Left/1(type) -> Bus Creator1/1
  A Straight B Left/2(resangle) -> Bus Creator1/2
  A Straight B Left/4(restime) -> Bus Creator1/4
  A Left B Straight/7(dphi_min) -> Bus Creator2/7
  A Left B Straight/6(tt_min) -> Bus Creator2/6
  Bus Creator2/1 -> Bus Creator4/3
  A Left B Straight/3(minsep) -> Bus Creator2/3
  A Left B Straight/5(dt_min) -> Bus Creator2/5
  A Left B Straight/1(type) -> Bus Creator2/1
  A Left B Straight/2(resangle) -> Bus Creator2/2
  A Left B Straight/4(restime) -> Bus Creator2/4
  A Right B Straight/7(dphi_min) -> Bus Creator3/7
  A Right B Straight/6(tt_min) -> Bus Creator3/6
  Bus Creator3/1 -> Bus Creator4/4
  A Right B Straight/3(minsep) -> Bus Creator3/3
  A Right B Straight/5(dt_min) -> Bus Creator3/5
  A Right B Straight/1(type) -> Bus Creator3/1
  A Right B Straight/2(resangle) -> Bus Creator3/2
  A Right B Straight/4(restime) -> Bus Creator3/4
  Bus Creator4/1 -> Std./1, To Workspace4/1

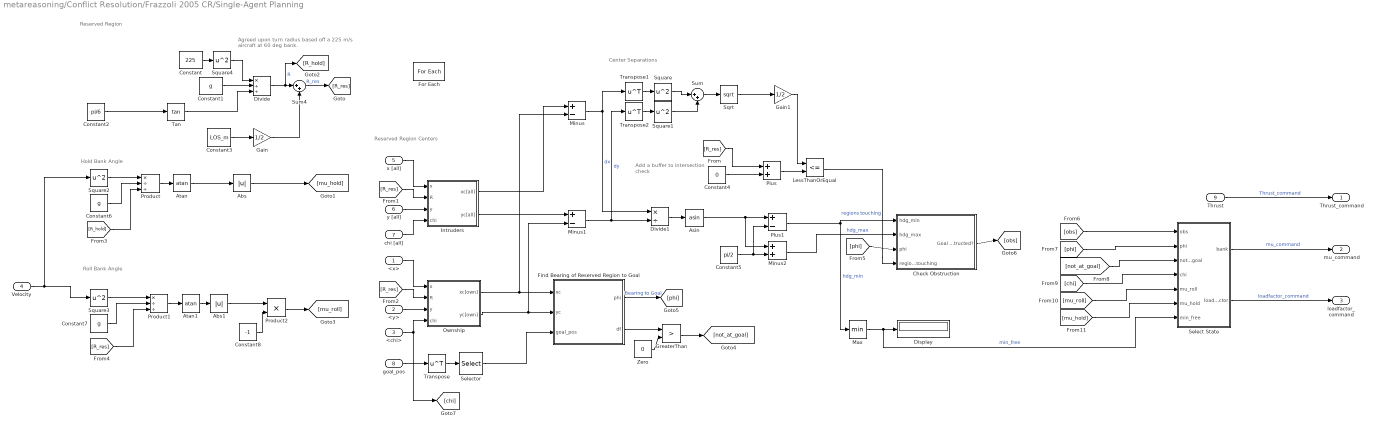
== system metareasoning/Conflict Resolution/Frazzoli 2005 CR/Single-Agent Planning ==
  note: Roll Bank Angle
  note: Hold Bank Angle
  note: Center Separations
  note: Reserved Region Centers
  note: Reserved Region
  note: Add a buffer to
      | intersection check
  note: Agreed upon turn radius based off a 225 m/s
      |  aircraft at 60 deg bank.
  <x> : Inport  Partition=on  PartitionDimension=1  PartitionWidth=1  PartitionOffset=0
  <y> : Inport  Port=2  Partition=on  PartitionDimension=1  PartitionWidth=1  PartitionOffset=0
  <chi> : Inport  Port=3  Partition=on  PartitionDimension=1  PartitionWidth=1  PartitionOffset=0
  Velocity : Inport  Port=4  Partition=on  PartitionDimension=1  PartitionWidth=1  PartitionOffset=0
  x [all] : Inport  Port=5
  y [all] : Inport  Port=6
  chi [all] : Inport  Port=7
  goal_pos : Inport  Port=8  Partition=on  PartitionDimension=1  PartitionWidth=1  PartitionOffset=0
  Thrust : Inport  Port=9  Partition=on  PartitionDimension=1  PartitionWidth=1  PartitionOffset=0
  Abs : Abs
  Abs1 : Abs
  Asin : Trigonometry  Operator=asin
  Atan : Trigonometry  Operator=atan
  Atan1 : Trigonometry  Operator=atan
  Check Obstruction : Subsystem
  Constant : Constant  Value=225
  Constant1 : Constant  Value=g
  Constant2 : Constant  Value=pi/6
  Constant3 : Constant  Value=LOS_m
  Constant4 : Constant  Value=0
  Constant5 : Constant  Value=pi/2
  Constant6 : Constant  Value=g
  Constant7 : Constant  Value=g
  Constant8 : Constant  Value=-1
  Display : Display
  Divide : Product  Inputs=*//
  Divide1 : Product  Inputs=*/
  Find Bearing of Reserved Region to Goal : MATLAB Function  TreatAsAtomicUnit=on
  For Each : ForEach  DisableCoverage=on
  Gain : Gain  Gain=1/2
  Gain1 : Gain  Gain=1/2
  GreaterThan : RelationalOperator  Operator=>  OutDataTypeStr=boolean  RndMeth=Simplest
  Intruders : Subsystem
  LessThanOrEqual : RelationalOperator  Operator=<=  OutDataTypeStr=boolean  RndMeth=Simplest
  Max : MinMax
  Minus : Sum  Inputs=+-
  Minus1 : Sum  Inputs=+-
  Minus2 : Sum
  Ownship : Subsystem
  Plus : Sum
  Plus1 : Sum  Inputs=+-
  Product : Product  Inputs=*//
  Product1 : Product  Inputs=*//
  Product2 : Product
  Select State : MATLAB Function  TreatAsAtomicUnit=on
  Selector : Selector  InputPortWidth=3  IndexOptions=Index vector (dialog)  Indices=[1 2]  OutputSizes=1
  Sqrt : Sqrt  SaturateOnIntegerOverflow=on
  Square{,1..4} (5 alike) : Math  Operator=square  SaturateOnIntegerOverflow=on
  Sum : Sum  Inputs=|++
  Sum4 : Sum  Inputs=|++
  Tan : Trigonometry  Operator=tan
  Transpose : Math  Operator=transpose  SaturateOnIntegerOverflow=on
  Transpose1 : Math  Operator=transpose  SaturateOnIntegerOverflow=on
  Transpose2 : Math  Operator=transpose  SaturateOnIntegerOverflow=on
  Zero : Constant  Value=0  OutDataTypeStr=Inherit: Inherit via back propagation
  Thrust_command : Outport  ConcatenationDimension=1
  mu_command : Outport  Port=2  ConcatenationDimension=1
  loadfactor_command : Outport  Port=3  ConcatenationDimension=1
  wires:
  LessThanOrEqual/1 -> Check Obstruction/4(regions touching)  "regions touching"
  Divide1/1 -> Asin/1
  Plus1/1 -> Max/1, Check Obstruction/1(hdg_min)  "hdg_min"
  [R_res] -> Plus/1
  Gain1/1 -> LessThanOrEqual/1
  Minus2/1 -> Check Obstruction/2(hdg_max)  "hdg_max"
  goal_pos/1 -> Transpose/1
  Constant4/1 -> Plus/2
  Plus/1 -> LessThanOrEqual/2
  Ownship/2(yc[own]) -> Minus1/2, Find Bearing of Reserved Region to Goal/2(yc)
  Transpose/1 -> Selector/1
  Selector/1 -> Find Bearing of Reserved Region to Goal/3(goal_pos)
  <x>/1 -> Ownship/1(x)
  Constant5/1 -> Minus2/2, Plus1/2
  <y>/1 -> Ownship/3(y)
  <chi>/1 -> [chi], Ownship/4(chi)
  x [all]/1 -> Intruders/1(x)
  y [all]/1 -> Intruders/3(y)
  chi [all]/1 -> Intruders/4(chi)
  [R_res] -> Intruders/2(R)
  Intruders/1(xc[all]) -> Minus/1
  Intruders/2(yc[all]) -> Minus1/1
  Constant1/1 -> Divide/2
  [R_res] -> Ownship/2(R)
  Asin/1 -> Minus2/1, Plus1/1
  Minus1/1 -> Divide1/2, Transpose2/1  "dy"
  Minus/1 -> Transpose1/1, Divide1/1  "dx"
  Ownship/1(xc[own]) -> Minus/2, Find Bearing of Reserved Region to Goal/1(xc)
  Sum4/1 -> [R_res]  "R_res"
  Constant3/1 -> Gain/1
  Gain/1 -> Sum4/2
  Divide/1 -> [R_hold], Sum4/1  "R"
  Tan/1 -> Divide/3
  Constant/1 -> Square4/1
  Constant2/1 -> Tan/1
  Transpose1/1 -> Square/1
  Transpose2/1 -> Square1/1
  Square/1 -> Sum/1
  Square1/1 -> Sum/2
  Sum/1 -> Sqrt/1
  Sqrt/1 -> Gain1/1
  Find Bearing of Reserved Region to Goal/1(phi) -> [phi]  "Bearing to Goal"
  Find Bearing of Reserved Region to Goal/2(df) -> GreaterThan/1
  [R_hold] -> Product/3
  Velocity/1 -> Square3/1, Square2/1
  Square2/1 -> Product/1
  Constant6/1 -> Product/2
  Product/1 -> Atan/1
  Atan/1 -> Abs/1
  [R_res] -> Product1/3
  Constant7/1 -> Product1/2
  Product1/1 -> Atan1/1
  Square3/1 -> Product1/1
  Abs1/1 -> Product2/1
  Atan1/1 -> Abs1/1
  Constant8/1 -> Product2/2
  Product2/1 -> [mu_roll]
  Max/1 -> Display/1, Select State/7(min_free)  "min_free"
  Check Obstruction/1(Goal Obstructed?) -> [obs]
  [phi] -> Check Obstruction/3(phi)
  Zero/1 -> GreaterThan/2
  GreaterThan/1 -> [not_at_goal]
  [not_at_goal] -> Select State/3(not_at_goal)
  [obs] -> Select State/1(obs)
  [mu_roll] -> Select State/5(mu_roll)
  [mu_hold] -> Select State/6(mu_hold)
  Thrust/1 -> Thrust_command/1  "Thrust_command"
  Select State/1(bank) -> mu_command/1  "mu_command"
  Select State/2(loadfactor) -> loadfactor_command/1  "loadfactor_command"
  [phi] -> Select State/2(phi)
  Square4/1 -> Divide/1
  [chi] -> Select State/4(chi)
  Abs/1 -> [mu_hold]

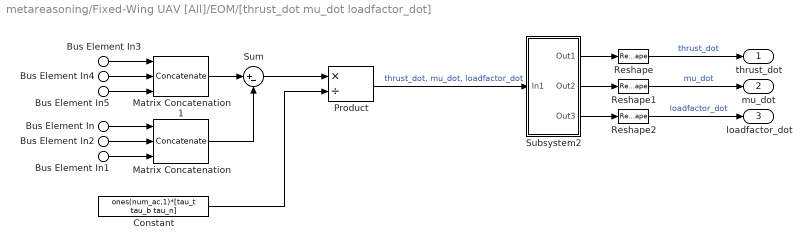
== system metareasoning/Fixed-Wing UAV [All]/EOM/[thrust_dot mu_dot loadfactor_dot] ==
  Bus Element In3 : Inport  PortName=Commands  Element=Thrust_command
  Bus Element In4 : Inport  PortName=Commands  Element=mu_command
  Bus Element In5 : Inport  PortName=Commands  Element=loadfactor_command
  Bus Element In : Inport  Port=2  PortName=States  Element=thrust
  Bus Element In1 : Inport  Port=2  PortName=States  Element=loadfactor
  Bus Element In2 : Inport  Port=2  PortName=States  Element=mu
  Constant : Constant  Value=ones(num_ac,1)*[tau_t tau_b tau_n]
  Matrix Concatenation : Concatenate  NumInputs=3  Mode=Multidimensional array  ConcatenateDimension=2
  Matrix Concatenation1 : Concatenate  NumInputs=3  Mode=Multidimensional array  ConcatenateDimension=2
  Product : Product  Inputs=*/  InputSameDT=on  SaturateOnIntegerOverflow=on  OutDataTypeStr=Inherit: Same as first input
  Reshape : Reshape
  Reshape1 : Reshape
  Reshape2 : Reshape
  Subsystem2 : Subsystem
      mask Display: disp('Select\nColumns');
  Sum : Sum  Inputs=|+-  InputSameDT=on  SaturateOnIntegerOverflow=on  OutDataTypeStr=Inherit: Same as first input
  thrust_dot : Outport  VectorParamsAs1DForOutWhenUnconnected=off
  mu_dot : Outport  Port=2  VectorParamsAs1DForOutWhenUnconnected=off
  loadfactor_dot : Outport  Port=3  VectorParamsAs1DForOutWhenUnconnected=off
  wires:
  Sum/1 -> Product/1
  Constant/1 -> Product/2
  Product/1 -> Subsystem2/1(In1)  "thrust_dot, mu_dot, loadfactor_dot"
  Subsystem2/1(Out1) -> Reshape/1
  Subsystem2/2(Out2) -> Reshape1/1
  Subsystem2/3(Out3) -> Reshape2/1
  Reshape/1 -> thrust_dot/1  "thrust_dot"
  Reshape1/1 -> mu_dot/1  "mu_dot"
  Reshape2/1 -> loadfactor_dot/1  "loadfactor_dot"
  Bus Element In/1 -> Matrix Concatenation/1
  Bus Element In2/1 -> Matrix Concatenation/2
  Bus Element In1/1 -> Matrix Concatenation/3
  Matrix Concatenation/1 -> Sum/2
  Bus Element In3/1 -> Matrix Concatenation1/1
  Bus Element In5/1 -> Matrix Concatenation1/3
  Bus Element In4/1 -> Matrix Concatenation1/2
  Matrix Concatenation1/1 -> Sum/1

== system metareasoning/Fixed-Wing UAV [All]/makebus1/Subsystem3 ==
  In1 : Inport
  Selector1 : Selector  NumberOfDimensions=2  InputPortWidth=3  IndexOptions=Index vector (dialog),Index vector (dialog)  Indices=1,1:num_ac  OutputSizes=1,1
  Selector2 : Selector  NumberOfDimensions=2  InputPortWidth=3  IndexOptions=Index vector (dialog),Index vector (dialog)  Indices=2,1:num_ac  OutputSizes=1,1
  Selector3 : Selector  NumberOfDimensions=2  InputPortWidth=3  IndexOptions=Index vector (dialog),Index vector (dialog)  Indices=3,1:num_ac  OutputSizes=1,1
  Out1 : Outport  VectorParamsAs1DForOutWhenUnconnected=off
  Out2 : Outport  Port=2  VectorParamsAs1DForOutWhenUnconnected=off
  Out3 : Outport  Port=3  VectorParamsAs1DForOutWhenUnconnected=off
  wires:
  Selector3/1 -> Out3/1
  In1/1 -> Selector2/1, Selector1/1, Selector3/1
  Selector1/1 -> Out1/1
  Selector2/1 -> Out2/1

== system metareasoning/Conflict Resolution/Erzberger 2010/Cooperative Maneuvers/A Left B Left ==
  d_ab : Inport
  Turn Radius : Inport  Port=2
  States : Inport  Port=3
  Time to Turn : Inport  Port=4
  Bus Selector : BusSelector  OutputSignals=x,y,Velocity,chi
  Constant : Constant  Value=turnangles(1:76)
  Find Resolution : MATLAB Function  TreatAsAtomicUnit=on
  "Select " : Selector  NumberOfDimensions=2  InputPortWidth=length(turnangles)  IndexOptions=Index vector (dialog),Index vector (dialog)  Indices=[1:76],1  OutputSizes=1,1
  Select Left Turn : Selector  InputPortWidth=length(turnangles)  IndexOptions=Index vector (dialog)  Indices=[1:76]  OutputSizes=1
  type : Outport
  resangle : Outport  Port=2
  minsep : Outport  Port=3
  restime : Outport  Port=4
  dt_min : Outport  Port=5
  tt_min : Outport  Port=6
  dphi_min : Outport  Port=7
  wires:
  "Select "/1 -> Find Resolution/6(tt)  "dt_aleft"
  Bus Selector/1 -> Find Resolution/1(x)  "<x>"
  States/1 -> Bus Selector/1
  d_ab/1 -> Select Left Turn/1
  Turn Radius/1 -> Find Resolution/7(R)  "R"
  Time to Turn/1 -> "Select "/1
  Select Left Turn/1 -> Find Resolution/5(dt)  "dt_aleft"
  Bus Selector/4 -> Find Resolution/4(chi)  "<chi>"
  Bus Selector/3 -> Find Resolution/3(V)  "<Velocity>"
  Constant/1 -> Find Resolution/8(angles)  "turnangles"
  Find Resolution/3(restime) -> restime/1
  Bus Selector/2 -> Find Resolution/2(y)  "<y>"
  Find Resolution/1(type) -> type/1
  Find Resolution/5(dt_min) -> dt_min/1
  Find Resolution/4(minsep) -> minsep/1
  Find Resolution/6(tt_min) -> tt_min/1
  Find Resolution/7(dphi_min) -> dphi_min/1
  Find Resolution/2(resangle) -> resangle/1

== system metareasoning/Conflict Resolution/Erzberger 2010/Cooperative Maneuvers/A Left B Right ==
  d_ab : Inport
  Turn Radius : Inport  Port=2
  States : Inport  Port=3
  Time to Turn : Inport  Port=4
  Bus Selector : BusSelector  OutputSignals=x,y,Velocity,chi
  Constant : Constant  Value=turnangles(1:76)
  Find Resolution : MATLAB Function  TreatAsAtomicUnit=on
  "Select " : Selector  NumberOfDimensions=2  InputPortWidth=length(turnangles)  IndexOptions=Index vector (dialog),Index vector (dialog)  Indices=[1:76],1  OutputSizes=1,1
  Select Right Turn : Selector  InputPortWidth=length(turnangles)  IndexOptions=Index vector (dialog)  Indices=[1:76]  OutputSizes=1
  type : Outport
  resangle : Outport  Port=2
  minsep : Outport  Port=3
  restime : Outport  Port=4
  dt_min : Outport  Port=5
  tt_min : Outport  Port=6
  dphi_min : Outport  Port=7
  wires:
  "Select "/1 -> Find Resolution/6(tt)  "dt_aleft"
  Bus Selector/1 -> Find Resolution/1(x)  "<x>"
  States/1 -> Bus Selector/1
  d_ab/1 -> Select Right Turn/1
  Turn Radius/1 -> Find Resolution/7(R)  "R"
  Time to Turn/1 -> "Select "/1
  Select Right Turn/1 -> Find Resolution/5(dt)  "dt_aleft"
  Bus Selector/4 -> Find Resolution/4(chi)  "<chi>"
  Bus Selector/3 -> Find Resolution/3(V)  "<Velocity>"
  Constant/1 -> Find Resolution/8(angles)  "turnangles"
  Find Resolution/3(restime) -> restime/1
  Bus Selector/2 -> Find Resolution/2(y)  "<y>"
  Find Resolution/1(type) -> type/1
  Find Resolution/5(dt_min) -> dt_min/1
  Find Resolution/4(minsep) -> minsep/1
  Find Resolution/6(tt_min) -> tt_min/1
  Find Resolution/7(dphi_min) -> dphi_min/1
  Find Resolution/2(resangle) -> resangle/1

== system metareasoning/Conflict Resolution/Erzberger 2010/Cooperative Maneuvers/A Right B Left ==
  d_ab : Inport
  Turn Radius : Inport  Port=2
  States : Inport  Port=3
  Time to Turn : Inport  Port=4
  Bus Selector : BusSelector  OutputSignals=x,y,Velocity,chi
  Constant : Constant  Value=turnangles(77:151)
  Find Resolution : MATLAB Function  TreatAsAtomicUnit=on
  "Select " : Selector  NumberOfDimensions=2  InputPortWidth=length(turnangles)  IndexOptions=Index vector (dialog),Index vector (dialog)  Indices=[77:151],1  OutputSizes=1,1
  Select Right Turn : Selector  InputPortWidth=length(turnangles)  IndexOptions=Index vector (dialog)  Indices=[77:151]  OutputSizes=1
  type : Outport
  resangle : Outport  Port=2
  minsep : Outport  Port=3
  restime : Outport  Port=4
  dt_min : Outport  Port=5
  tt_min : Outport  Port=6
  dphi_min : Outport  Port=7
  wires:
  "Select "/1 -> Find Resolution/6(tt)  "dt_aright"
  Bus Selector/1 -> Find Resolution/1(x)  "<x>"
  States/1 -> Bus Selector/1
  d_ab/1 -> Select Right Turn/1
  Turn Radius/1 -> Find Resolution/7(R)  "R"
  Time to Turn/1 -> "Select "/1
  Select Right Turn/1 -> Find Resolution/5(dt)  "dt_aright"
  Bus Selector/4 -> Find Resolution/4(chi)  "<chi>"
  Bus Selector/3 -> Find Resolution/3(V)  "<Velocity>"
  Constant/1 -> Find Resolution/8(angles)  "turnangles"
  Find Resolution/3(restime) -> restime/1
  Bus Selector/2 -> Find Resolution/2(y)  "<y>"
  Find Resolution/1(type) -> type/1
  Find Resolution/5(dt_min) -> dt_min/1
  Find Resolution/4(minsep) -> minsep/1
  Find Resolution/6(tt_min) -> tt_min/1
  Find Resolution/7(dphi_min) -> dphi_min/1
  Find Resolution/2(resangle) -> resangle/1

== system metareasoning/Conflict Resolution/Erzberger 2010/Cooperative Maneuvers/A Right B Right ==
  d_ab : Inport
  Turn Radius : Inport  Port=2
  States : Inport  Port=3
  Time to Turn : Inport  Port=4
  Bus Selector : BusSelector  OutputSignals=x,y,Velocity,chi
  Constant : Constant  Value=turnangles(77:151)
  Find Resolution : MATLAB Function  TreatAsAtomicUnit=on
  "Select " : Selector  NumberOfDimensions=2  InputPortWidth=length(turnangles)  IndexOptions=Index vector (dialog),Index vector (dialog)  Indices=[77:151],1  OutputSizes=1,1
  Select Right Turn : Selector  InputPortWidth=length(turnangles)  IndexOptions=Index vector (dialog)  Indices=[77:151]  OutputSizes=1
  type : Outport
  resangle : Outport  Port=2
  minsep : Outport  Port=3
  restime : Outport  Port=4
  dt_min : Outport  Port=5
  tt_min : Outport  Port=6
  dphi_min : Outport  Port=7
  wires:
  "Select "/1 -> Find Resolution/6(tt)  "dt_aright"
  Bus Selector/1 -> Find Resolution/1(x)  "<x>"
  States/1 -> Bus Selector/1
  d_ab/1 -> Select Right Turn/1
  Turn Radius/1 -> Find Resolution/7(R)  "R"
  Time to Turn/1 -> "Select "/1
  Select Right Turn/1 -> Find Resolution/5(dt)  "dt_aright"
  Bus Selector/4 -> Find Resolution/4(chi)  "<chi>"
  Bus Selector/3 -> Find Resolution/3(V)  "<Velocity>"
  Constant/1 -> Find Resolution/8(angles)  "turnangles"
  Find Resolution/3(restime) -> restime/1
  Bus Selector/2 -> Find Resolution/2(y)  "<y>"
  Find Resolution/1(type) -> type/1
  Find Resolution/5(dt_min) -> dt_min/1
  Find Resolution/4(minsep) -> minsep/1
  Find Resolution/6(tt_min) -> tt_min/1
  Find Resolution/7(dphi_min) -> dphi_min/1
  Find Resolution/2(resangle) -> resangle/1

== system metareasoning/Conflict Resolution/Erzberger 2010/Cooperative Maneuvers/Time To Turn ==
  Velocity : Inport
  Abs : Abs
  Constant : Constant  Value=g
  Constant1 : Constant  Value=tand(30)
  Divide : Product  Inputs=*//
  Matrix Multiply : Product  Multiplication=Matrix(*)
  Reshape : Reshape  OutputDimensionality=Row vector (2-D)
  Turn Angles : Constant  Value=turnangles  VectorParams1D=off
  Time to Turn : Outport
  wires:
  Constant1/1 -> Divide/3
  Divide/1 -> Reshape/1
  Matrix Multiply/1 -> Abs/1
  Reshape/1 -> Matrix Multiply/2
  Velocity/1 -> Divide/1
  Constant/1 -> Divide/2
  Turn Angles/1 -> Matrix Multiply/1
  Abs/1 -> Time to Turn/1

== system metareasoning/Conflict Resolution/Erzberger 2010/Cooperative Maneuvers/Turn Radius (2) ==
  States : Inport
  Bus Selector : BusSelector  OutputSignals=Velocity
  Constant : Constant  Value=g*tan(deg2rad(30))
  Divide : Product  Inputs=*/
  Square : Math  Operator=square  SaturateOnIntegerOverflow=on
  Turn Radius : Outport
  wires:
  Divide/1 -> Turn Radius/1
  States/1 -> Bus Selector/1
  Constant/1 -> Divide/2
  Square/1 -> Divide/1
  Bus Selector/1 -> Square/1  "<Velocity>"

== system metareasoning/Conflict Resolution/Erzberger 2010/Cooperative Maneuvers/d_ab b left(13) ==
  States : Inport
  Turn Radius : Inport  Port=2
  Bus Selector : BusSelector  OutputSignals=Velocity,chi,x,y
  d_ab b left (13) : MATLAB Function  TreatAsAtomicUnit=on
  d_ab B left : Outport
  wires:
  Bus Selector/4 -> d_ab b left (13)/4(y)  "<y>"
  Bus Selector/2 -> d_ab b left (13)/2(chi)  "<chi>"
  d_ab b left (13)/1(d_ab) -> d_ab B left/1
  Bus Selector/3 -> d_ab b left (13)/3(x)  "<x>"
  Bus Selector/1 -> d_ab b left (13)/1(v)  "<Velocity>"
  Turn Radius/1 -> d_ab b left (13)/5(R)
  States/1 -> Bus Selector/1
